simulink model "sdf_target"  (R2020a)
settings: Solver=FixedStepAuto  StartTime=0.0  StopTime=inf  FixedStep=0.01  RelTol=1e-3  EnableMultiTasking=on
undefined symbols (not defined in the file or in its folder): DiscIntNeverNeededParam, X, Y, Z
libraries: robotlib x6, sensehatlib x1
settings Model: SimulationMode=external  Creator=HannesDittmann  LastModifiedBy=alf
settings SolverCC: PositivePriorityOrder=on
settings DataIOCC: ReturnWorkspaceOutputs=off
settings OptimizationCC: EnhancedBackFolding=on  PassReuseOutputArgsAs=Individual arguments  MaxStackSize=64  OptimizeBlockOrder=speed  DifferentSizesBufferReuse=on  OptimizationCustomize=off  EfficientTunableParamExpr=on
settings DebuggingCC: ParameterTunabilityLossMsg=error  ArithmeticOperatorsInVariantConditions=warning
settings HardwareCC: ProdBitPerPointer=32  ProdBitPerSizeT=32  ProdBitPerPtrDiffT=32  ProdLargestAtomicInteger=Long  ProdLargestAtomicFloat=Double  ProdWordSize=32  ProdHWDeviceType=ARM Compatible->ARM Cortex
settings SFSimCC: CustomCodeUndefinedFunction=UseInterfaceOnly
settings RTWCC: SystemTargetFile=ert.tlc  HardwareBoard=Raspberry Pi - Robot Operating System (ROS)  TemplateMakefile=ert_default_tmf  GenerateReport=on  Toolchain=Catkin  BuildConfiguration=Faster Runs  IncludeHyperlinkInReport=on  LaunchReport=on  TargetLang=C++  GenerateTraceInfo=on  GenerateTraceReport=on  GenerateTraceReportSl=on  GenerateTraceReportSf=on  GenerateTraceReportEml=on
settings CodeAppCC: ForceParamTrailComments=on  IgnoreCustomStorageClasses=off  OperatorAnnotations=on  SimulinkDataObjDesc=on  SFDataObjDesc=on  InsertBlockDesc=on
settings ERTTargetCC: SupportContinuousTime=on  SupportVariableSizeSignals=on  ExtMode=on  ExtModeMexArgs='192.168.1.6' 0 17725

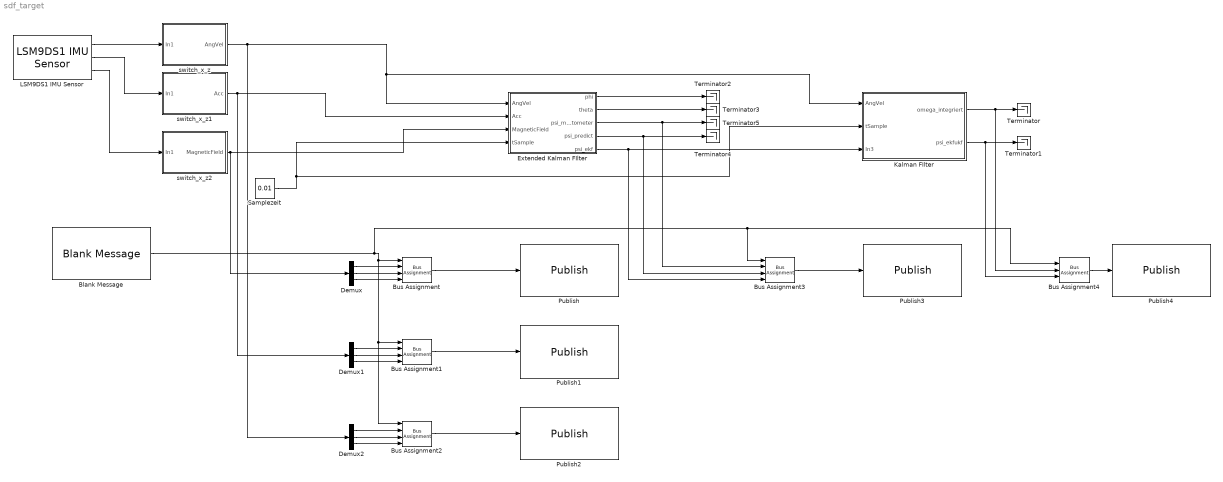
== system sdf_target ==
  Blank Message : robotlib/Blank Message  messageClass=Message  entityType=geometry_msgs/Point  messageType=geometry_msgs/Point  SampleTime=-1
  Bus Assignment{,1..3} (4 alike) : BusAssignment  AssignedSignals=X,Y,Z
  Bus Assignment4 : BusAssignment  AssignedSignals=Y,Z
  Demux : Demux  Outputs=3
  Demux1 : Demux  Outputs=3
  Demux2 : Demux  Outputs=3
  Extended Kalman FIlter : Subsystem
  Kalman FIlter : Subsystem
  LSM9DS1 IMU Sensor : sensehatlib/LSM9DS1 IMU Sensor  blockPlatform=Raspberry Pi  BoardProperty_sh=Model B+  ActiveSensors_=Accelerometer, Gyroscope and Magnetometer  AccelerometerOutputDataRate=119 Hz  AccelerometerFullScaleRange=+/- 2g  AccelerometerBandwidth=50 Hz  GyroscopeOutputDataRate=119 Hz  GyroscopeFullScaleRange=245 dps  GyroscopeBandwidthMode=0  GyroscopeHighPassFilterEnabled=off  GyroscopeHighPassFilterMode=0  MagnetometerFullScaleRange=+/- 4 gauss  MagnetometerOutputDataRate=40 Hz  SampleTime=0.01
      settings: SourceProductBaseCode=RASPPI
  Publish : robotlib/Publish  topicSource=Specify your own  topic=/mag_lsm9ds1  messageType=geometry_msgs/Point  messageQueueLength=1
  Publish1 : robotlib/Publish  topicSource=Specify your own  topic=/accel_lsm9ds1  messageType=geometry_msgs/Point  messageQueueLength=1
  Publish2 : robotlib/Publish  topicSource=Specify your own  topic=/angVel_lsm9ds1  messageType=geometry_msgs/Point  messageQueueLength=1
  Publish3 : robotlib/Publish  topicSource=Specify your own  topic=/psi_ekf  messageType=geometry_msgs/Point  messageQueueLength=1
  Publish4 : robotlib/Publish  topicSource=Specify your own  topic=/psi_ekf_kf  messageType=geometry_msgs/Point  messageQueueLength=1
  Samplezeit : Constant  Value=0.01
  Terminator{,1..5} (6 alike) : Terminator
  switch_x_z : Subsystem
  switch_x_z1 : Subsystem
  switch_x_z2 : Subsystem
  wires:
  Samplezeit/1 -> Extended Kalman FIlter/4(tSample), Kalman FIlter/2(tSample)
  Extended Kalman FIlter/5(psi_ekf) -> Bus Assignment3/4, Kalman FIlter/3(In3)
  Extended Kalman FIlter/1(phi) -> Terminator2/1
  Extended Kalman FIlter/2(theta) -> Terminator3/1
  LSM9DS1 IMU Sensor/1 -> switch_x_z/1(In1)
  LSM9DS1 IMU Sensor/2 -> switch_x_z1/1(In1)
  LSM9DS1 IMU Sensor/3 -> switch_x_z2/1(In1)
  switch_x_z/1(AngVel) -> Extended Kalman FIlter/1(AngVel), Kalman FIlter/1(AngVel), Demux2/1
  switch_x_z1/1(Acc) -> Demux1/1, Extended Kalman FIlter/2(Acc)
  switch_x_z2/1(MagneticField) -> Demux/1, Extended Kalman FIlter/3(MagneticField)
  Kalman FIlter/1(omega_integriert) -> Bus Assignment4/2, Terminator/1
  Kalman FIlter/2(psi_ekfukf) -> Bus Assignment4/3, Terminator1/1
  Extended Kalman FIlter/4(psi_predict) -> Bus Assignment3/3, Terminator4/1
  Bus Assignment/1 -> Publish/1
  Demux/1 -> Bus Assignment/2
  Demux/2 -> Bus Assignment/3
  Demux/3 -> Bus Assignment/4
  Blank Message/1 -> Bus Assignment4/1, Bus Assignment3/1, Bus Assignment2/1, Bus Assignment1/1, Bus Assignment/1
  Bus Assignment1/1 -> Publish1/1
  Demux1/1 -> Bus Assignment1/2
  Demux1/2 -> Bus Assignment1/3
  Demux1/3 -> Bus Assignment1/4
  Bus Assignment2/1 -> Publish2/1
  Demux2/1 -> Bus Assignment2/2
  Demux2/2 -> Bus Assignment2/3
  Demux2/3 -> Bus Assignment2/4
  Extended Kalman FIlter/3(psi_magnetometer) -> Bus Assignment3/2, Terminator5/1
  Bus Assignment3/1 -> Publish3/1
  Bus Assignment4/1 -> Publish4/1

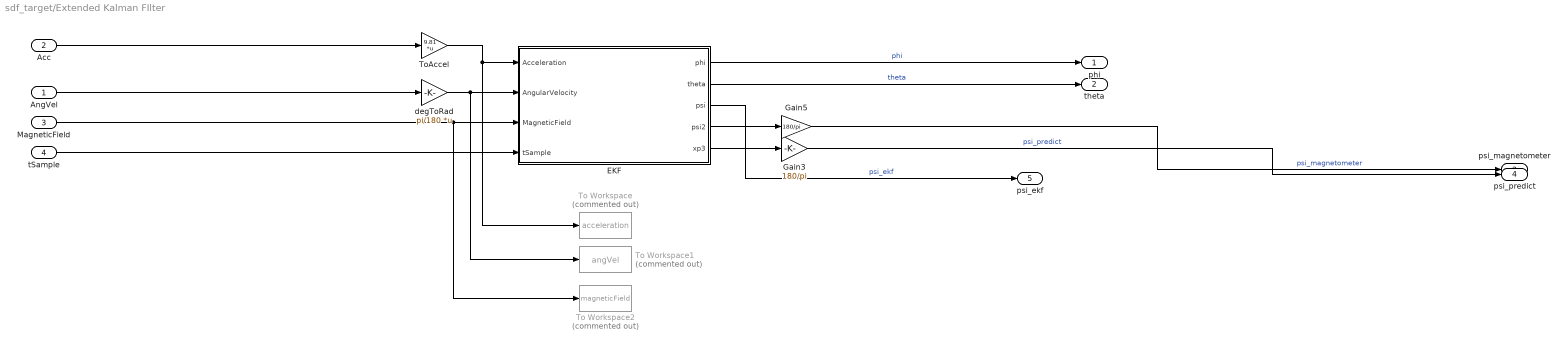
== system sdf_target/Extended Kalman FIlter ==
  AngVel : Inport
  Acc : Inport  Port=2
  MagneticField : Inport  Port=3
  tSample : Inport  Port=4
  EKF : MATLAB Function  TreatAsAtomicUnit=on
  Gain3 : Gain  Gain=180/pi
  Gain5 : Gain  Gain=180/pi
  To Workspace : ToWorkspace  Commented=on  VariableName=acceleration  SampleTime=-1
  To Workspace1 : ToWorkspace  Commented=on  VariableName=angVel  SampleTime=-1
  To Workspace2 : ToWorkspace  Commented=on  VariableName=magneticField  SampleTime=-1
  ToAccel : Gain  Gain=9.81  Multiplication=Matrix(K*u)
  degToRad : Gain  Gain=pi/180  Multiplication=Matrix(K*u)
  phi : Outport  VectorParamsAs1DForOutWhenUnconnected=off
  theta : Outport  Port=2  VectorParamsAs1DForOutWhenUnconnected=off
  psi_magnetometer : Outport  Port=3  VectorParamsAs1DForOutWhenUnconnected=off
  psi_predict : Outport  Port=4  VectorParamsAs1DForOutWhenUnconnected=off
  psi_ekf : Outport  Port=5  VectorParamsAs1DForOutWhenUnconnected=off
  wires:
  EKF/1(phi) -> phi/1  "phi"
  tSample/1 -> EKF/4(tSample)
  Acc/1 -> ToAccel/1
  Gain3/1 -> psi_predict/1  "psi_predict"
  MagneticField/1 -> To Workspace2/1, EKF/3(MagneticField)
  EKF/5(xp3) -> Gain3/1
  EKF/3(psi) -> psi_ekf/1  "psi_ekf"
  degToRad/1 -> To Workspace1/1, EKF/2(AngularVelocity)
  EKF/4(psi2) -> Gain5/1
  Gain5/1 -> psi_magnetometer/1  "psi_magnetometer"
  EKF/2(theta) -> theta/1  "theta"
  AngVel/1 -> degToRad/1
  ToAccel/1 -> EKF/1(Acceleration), To Workspace/1

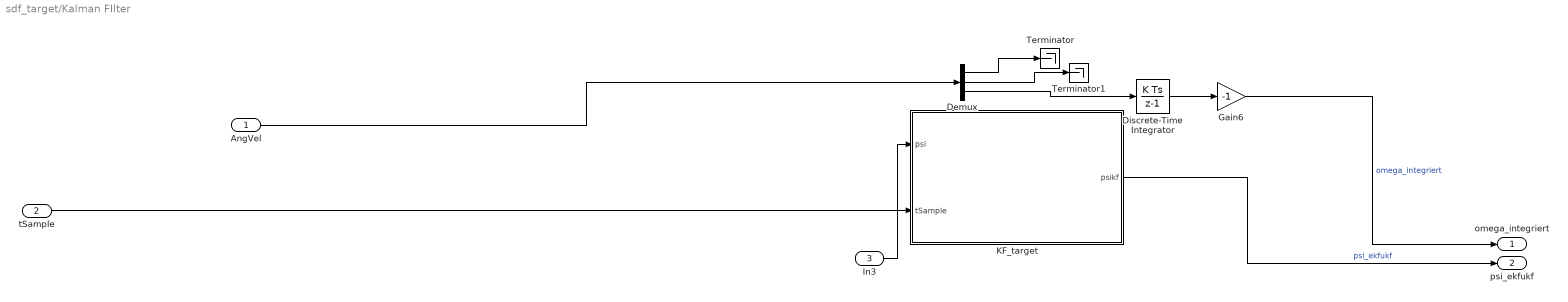
== system sdf_target/Kalman FIlter ==
  AngVel : Inport
  tSample : Inport  Port=2
  In3 : Inport  Port=3
  Demux : Demux  Outputs=3
  Discrete-Time Integrator : DiscreteIntegrator  SampleTime=-1  ICPrevOutput=DiscIntNeverNeededParam  ICPrevScaledInput=DiscIntNeverNeededParam
  Gain6 : Gain  Gain=-1
  KF_target : MATLAB Function  TreatAsAtomicUnit=on
  Terminator : Terminator
  Terminator1 : Terminator
  omega_integriert : Outport  VectorParamsAs1DForOutWhenUnconnected=off
  psi_ekfukf : Outport  Port=2  VectorParamsAs1DForOutWhenUnconnected=off
  wires:
  tSample/1 -> KF_target/2(tSample)
  In3/1 -> KF_target/1(psi)
  Gain6/1 -> omega_integriert/1  "omega_integriert"
  Demux/2 -> Terminator1/1
  KF_target/1(psikf) -> psi_ekfukf/1  "psi_ekfukf"
  Demux/3 -> Discrete-Time Integrator/1
  AngVel/1 -> Demux/1
  Demux/1 -> Terminator/1
  Discrete-Time Integrator/1 -> Gain6/1

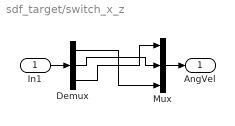
== system sdf_target/switch_x_z ==
  In1 : Inport
  Demux : Demux  Outputs=3
  Mux : Mux  Inputs=3
  AngVel : Outport
  wires:
  In1/1 -> Demux/1
  Demux/2 -> Mux/2
  Mux/1 -> AngVel/1
  Demux/1 -> Mux/3
  Demux/3 -> Mux/1

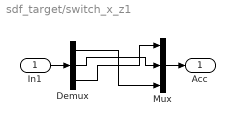
== system sdf_target/switch_x_z1 ==
  In1 : Inport
  Demux : Demux  Outputs=3
  Mux : Mux  Inputs=3
  Acc : Outport
  wires:
  Demux/3 -> Mux/1
  Demux/1 -> Mux/3
  Mux/1 -> Acc/1
  Demux/2 -> Mux/2
  In1/1 -> Demux/1

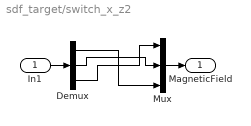
== system sdf_target/switch_x_z2 ==
  In1 : Inport
  Demux : Demux  Outputs=3
  Mux : Mux  Inputs=3
  MagneticField : Outport
  wires:
  In1/1 -> Demux/1
  Demux/2 -> Mux/2
  Mux/1 -> MagneticField/1
  Demux/1 -> Mux/3
  Demux/3 -> Mux/1

== matlab function sdf_target/Kalman FIlter/KF_target ==
  settings: updateMethod=DISCRETE
  data: psi input; psikf output; tSample input
function psikf   = fcn(psi,tSample)

persistent x_dach P Q R C I A_d firstRun

if isempty(firstRun)
    
  firstRun = 1;
  
     I=eye(2);

     A_d = [1.0000    0.0100;
           0    1.0000];
       
    C=[1 0];

    Q=0.001*I;

    R=1;

    P = 0.1*eye(2);

    x_dach = [psi 0]'; % Startwerte phi theta psi

end


%% Kalman Filter


xp = A_d*x_dach;

Pp = A_d*P*A_d' + Q;    

K = Pp*C'*inv(C*Pp*C' + R);

x_dach = xp + K*(psi - C*xp);

P = Pp - K*C*Pp;

psikf=x_dach(1);

end

== matlab function sdf_target/Extended Kalman FIlter/EKF ==
  settings: updateMethod=DISCRETE
  data: Acceleration input; phi output; AngularVelocity input; MagneticField input; tSample input; theta output; psi output; psi2 output; xp3 output
function [phi,theta,psi,psi2,xp3] = fcn(Acceleration,AngularVelocity,MagneticField,tSample)

%Funktion schaetzt die WInkel phi theta und psi mithilfe eines
%Extenden-Kalman Filters
%Eingabewerte: Daten aus LSM9DS1 fuer Sensordatenfusion und Samplezeit der
%form 3x1
%Ausgabewerte: WInkelschaetzungen phi, theta und psi sowie psi Berechnung
%durch Magnetometer und Praediktion des Winkels Psi aus dem EKF

persistent x_dach P Q R C I

persistent firstRun

if isempty(firstRun)
  firstRun = 1;
  
    I=eye(3); % EInheitsmatrix

    C=I;
  
%% Filtereinstellungen
    
    P = 0.01*I;


    Q=[.0001 0 0;
       0 .0001 0;       % Modellrauschen
       0 0 0.1];

    R=[1.9 0 0;
       0 1.82 0;        % Messrauschen
       0 0 11];

    x_dach = [0 0 0]'; % Startwerte phi theta psi

end


%% Extended-Kalman Filter

A_d = Ajacob(x_dach,AngularVelocity,tSample,I);     %Berechnung Jacobi-Matrix

[phi,theta,psi] = EulerAccel(x_dach, Acceleration(1),Acceleration(2),MagneticField); % Berechnung Messvektor 

[xp1,xp2,xp3] = fx(x_dach,AngularVelocity,tSample);     % Praediktion

Pp = A_d*P*A_d' + Q;                                    

K = Pp*C'*inv(C*Pp*C' + R);                             % Kalman-Verstaerkung

x_dach = [xp1 xp2 xp3]' + K*([phi theta psi]' - C*[xp1 xp2 xp3]'); % Korrektur des Zustandsvektor
P = Pp - K*C*Pp;


%% Ausgabe der Werte

psi2=psi;
phi=x_dach(1)*180/pi;
theta=x_dach(2)*180/pi;
psi=x_dach(3)*180/pi;

end

%% Funktion zur Berechnung der Messwerte

function [phi,theta,psi] = EulerAccel(x_dach,ax, ay, magnet)
%
%
g = 9.81; % Erdbeschleunigung in m/(s^2)

% Rückgabewerte sind die Eulerwinkel
theta = asin(  ax / g  );
phi   = asin( -ay /(g*cos(theta)));

xm=magnet(1);
ym=magnet(2);
zm=magnet(3);

xh = xm*cos(-x_dach(2))+zm*sin(-x_dach(2));
yh = xm*sin(-x_dach(1))*sin(-x_dach(2))+ym*cos(-x_dach(1))-zm*sin(-x_dach(1))*cos(-x_dach(2));


psi = mod(atan2(yh,xh),2*pi);

if psi < 0
    psi = psi + 2*pi;
end

end

%% Funktion zur Berechnung der Praediktion

function [xp1 xp2 xp3] = fx(xhat, rates, dt)
%
%
phi   = xhat(1);
theta = xhat(2);

p = rates(1);
q = rates(2);
r = rates(3);

xdot = zeros(3, 1);

xdot(1) = p + q*sin(phi)*tan(theta) + r*cos(phi)*tan(theta);
xdot(2) =     q*cos(phi)            - r*sin(phi);
xdot(3) =     q*sin(phi)/cos(theta) + r*cos(phi)/cos(theta);

xp1 = xhat(1) + xdot(1)*dt; % Prädiktion des Zustandsvektors
xp2 = xhat(2) + xdot(2)*dt;
xp3 = xhat(3) + xdot(3)*dt;

end


%% Jacobi-Matrix

function A = Ajacob(xhat, rates, dt,I)


A = zeros(3, 3);

phi   = xhat(1);
theta = xhat(2);

p = rates(1);
q = rates(2);
r = rates(3);

A(1,1) = q*cos(phi)*tan(theta)   - r*sin(phi)*tan(theta);
A(1,2) = q*sin(phi)/cos(theta)^2 + r*cos(phi)/cos(theta)^2;
A(1,3) = 0;

A(2,1) = -q*sin(phi) - r*cos(phi);
A(2,2) = 0;
A(2,3) = 0;

A(3,1) = q*cos(phi)/cos(theta) - r*sin(phi)/cos(theta);
A(3,2) = q*sin(phi)*sin(theta)/(2*cos(theta)^2) + r*cos(phi)*sin(theta)/(2*cos(theta));
A(3,3) = 0;

A = I+A*dt; % Linearisierung im AP
end
